simulink subsystem "Control_sub"  (R2023b)
settings: Solver=VariableStepAuto  StartTime=0.0  StopTime=10.0  RelTol=1e-3
libraries: Autonomous_lib x1, Disabled_lib x1, Swerve_Drive_lib x1, Teleop_lib x1, Test_lib x1
settings Model: Creator=USER  LastModifiedBy=USER

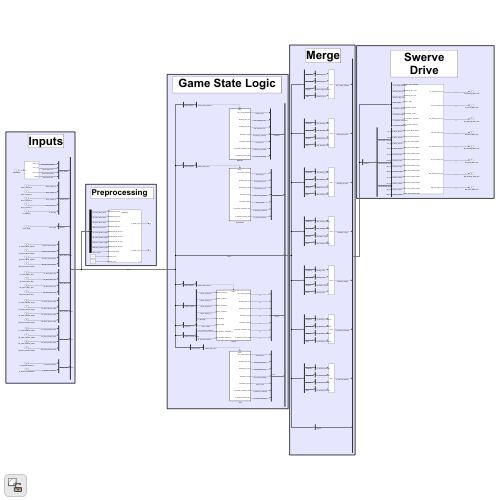
[thumbnail: Simulink's stored preview of the top-level diagram]
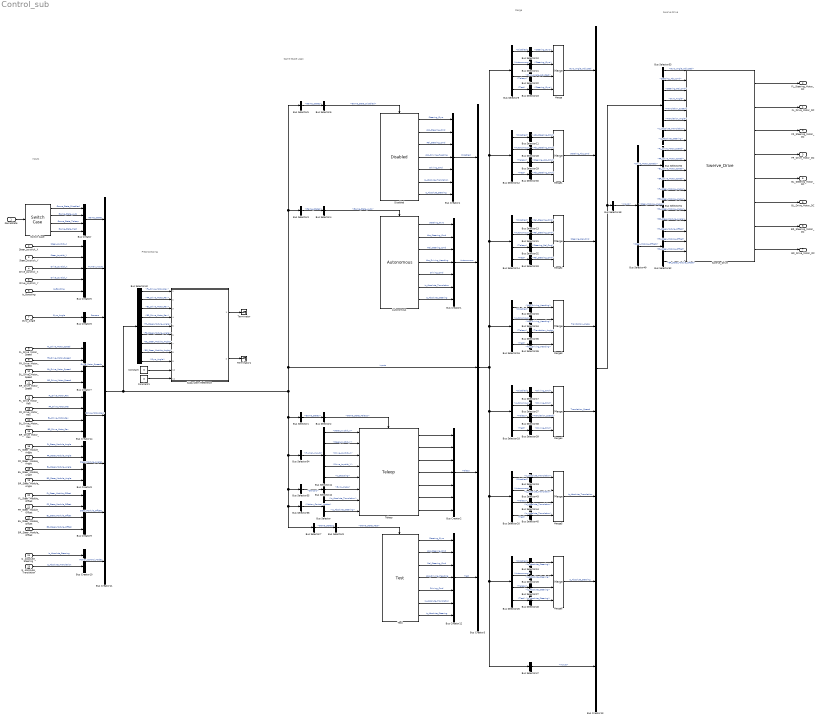
== system Control_sub ==
  note: Game State Logic
  note: Merge
  note: Swerve Drive
  note: Inputs
  note: Preprocessing
  GameState : Inport
  Steer_Joystick_X : Inport  Port=2
  Steer_Joystick_Y : Inport  Port=3
  Drive_Joystick_X : Inport  Port=4
  Drive_Joystick_Y : Inport  Port=5
  Is_Boosting : Inport  Port=6
  Gyro_Angle : Inport  Port=7
  FL_Drive_Motor_Speed : Inport  Port=8
  FR_Drive_Motor_Speed : Inport  Port=9
  BL_Drive_Motor_Speed : Inport  Port=10
  BR_Drive_Motor_Speed : Inport  Port=11
  FL_Drive_Motor_Rev : Inport  Port=12
  FR_Drive_Motor_Rev : Inport  Port=13
  BL_Drive_Motor_Rev : Inport  Port=14
  BR_Drive_Motor_Rev : Inport  Port=15
  FL_Steer_Module_Angle : Inport  Port=16
  FR_Steer_Module_Angle : Inport  Port=17
  BL_Steer_Module_Angle : Inport  Port=18
  BR_Steer_Module_Angle : Inport  Port=19
  FL_Steer_Module_Offset : Inport  Port=20
  FR_Steer_Module_Offset : Inport  Port=21
  BL_Steer_Module_Offset : Inport  Port=22
  BR_Steer_Module_Offset : Inport  Port=23
  Is_Absolute_Steering : Inport  Port=24
  Is_Absolute_Translation : Inport  Port=25
  Autonomous : Autonomous_lib/Autonomous  SystemSampleTime=-1  VariantActivationTime=update diagram  AllowFlexibleInterface=on  Latency=0  AutoFrameSizeCalculation=off
  Bus Creator{,7..9,14} (5 alike) : BusCreator  Inputs=4
  Bus Creator{1..2,4,12} (4 alike) : BusCreator  Inputs=7
  Bus Creator10 : BusCreator  Inputs=2
  Bus Creator11 : BusCreator  Inputs=8
  Bus Creator13 : BusCreator  Inputs=8
  Bus Creator3 : BusCreator  Inputs=5
  Bus Creator5 : BusCreator  Inputs=5
  Bus Creator6 : BusCreator  Inputs=1
  Bus Selector : BusSelector  OutputSignals=Is_Absolute_Translation,Is_Absolute_Steering
  Bus Selector{1,3,5,7} (4 alike) : BusSelector  OutputSignals=Game_States
  Bus Selector10 : BusSelector  OutputSignals=Steering_Gyro
  Bus Selector11 : BusSelector  OutputSignals=Abs_Steering_Cmd
  Bus Selector{9,12,14,16,18,20,25} (7 alike) : BusSelector  OutputSignals=Disabled,Autonomous,Teleop,Test
  Bus Selector13 : BusSelector  OutputSignals=Rel_Steering_Cmd
  Bus Selector15 : BusSelector  OutputSignals=Abs_Driving_Heading
  Bus Selector17 : BusSelector  OutputSignals=Driving_Cmd
  Bus Selector{19,43..45} (4 alike) : BusSelector  OutputSignals=Is_Absolute_Translation
  Bus Selector2 : BusSelector  OutputSignals=Game_State_Teleop
  Bus Selector21 : BusSelector  OutputSignals=Steering_Gyro
  Bus Selector22 : BusSelector  OutputSignals=Gyro_Angle_Adjusted
  Bus Selector23 : BusSelector  OutputSignals=Steering_Gyro
  Bus Selector{24,26..27,46} (4 alike) : BusSelector  OutputSignals=Is_Absolute_Steering
  Bus Selector28 : BusSelector  OutputSignals=Abs_Steering_Cmd
  Bus Selector29 : BusSelector  OutputSignals=Steering_Abs_Cmd
  Bus Selector30 : BusSelector  OutputSignals=Abs_Steering_Cmd
  Bus Selector31 : BusSelector  OutputSignals=Rel_Steering_Cmd
  Bus Selector32 : BusSelector  OutputSignals=Steering_Rel_Cmd
  Bus Selector33 : BusSelector  OutputSignals=Rel_Steering_Cmd
  Bus Selector34 : BusSelector  OutputSignals=Abs_Driving_Heading
  Bus Selector35 : BusSelector  OutputSignals=Translation_Angle
  Bus Selector36 : BusSelector  OutputSignals=Abs_Driving_Heading
  Bus Selector37 : BusSelector  OutputSignals=Driving_Cmd
  Bus Selector38 : BusSelector  OutputSignals=Translation_Speed
  Bus Selector39 : BusSelector  OutputSignals=Driving_Cmd
  Bus Selector4 : BusSelector  OutputSignals=Game_State_Auto
  Bus Selector40 : BusSelector  OutputSignals=Drive_Motor_Revs.FL_Drive_Motor_Rev,Drive_Motor_Revs.FR_Drive_Motor_Rev,Drive_Motor_Revs.BL_Drive_Motor_Rev,Drive_Motor_Revs.BR_Drive_Motor_Rev,Steer_Module_Angles.FL_Steer_Module_Angle,Steer_Module_Angles.FR_Steer_Module_Angle,Steer_Module_Angles.BL_Steer_Module_Angle,Steer_Module_Angles.BR_Steer_Module_Angle,Sensors.Gyro_Angle
  Bus Selector41 : BusSelector  OutputSignals=Steer_Joystick_X,Steer_Joystick_Y,Drive_Joystick_X,Drive_Joystick_Y,Is_Boosting
  Bus Selector42 : BusSelector  OutputSignals=Gyro_Angle
  Bus Selector47 : BusSelector  OutputSignals=Inputs
  Bus Selector48 : BusSelector  OutputSignals=Inputs
  Bus Selector49 : BusSelector  OutputSignals=Drive_Motor_Speeds,Steer_Module_Angles,Steer_Module_Offsets
  Bus Selector50 : BusSelector  OutputSignals=FL_Drive_Motor_Speed,FR_Drive_Motor_Speed,BL_Drive_Motor_Speed,BR_Drive_Motor_Speed
  Bus Selector51 : BusSelector  OutputSignals=FL_Steer_Module_Angle,FR_Steer_Module_Angle,BL_Steer_Module_Angle,BR_Steer_Module_Angle
  Bus Selector52 : BusSelector  OutputSignals=FL_Steer_Module_Offset,FR_Steer_Module_Offset,BL_Steer_Module_Offset,BR_Steer_Module_Offset
  Bus Selector53 : BusSelector  OutputSignals=Gyro_Angle_Adjusted,Steering_Abs_Cmd,Steering_Rel_Cmd,Inputs.Sensors.Gyro_Angle,Translation_Speed,Translation_Angle,Is_Absolute_Translation,Is_Absolute_Steering
  Bus Selector54 : BusSelector  OutputSignals=Human_Inputs
  Bus Selector55 : BusSelector  OutputSignals=Sensors
  Bus Selector56 : BusSelector  OutputSignals=Motion_Control_Modes
  Bus Selector6 : BusSelector  OutputSignals=Game_State_Disabled
  Bus Selector8 : BusSelector  OutputSignals=Game_State_Test
  Constant : Constant  Value=0
  Constant1 : Constant  Value=0
  Disabled : Disabled_lib/Disabled  SystemSampleTime=-1  VariantActivationTime=update diagram  AllowFlexibleInterface=on  Latency=0  AutoFrameSizeCalculation=off
  Merge{,1..6} (7 alike) : Merge  Inputs=4
  Subsystem Reference : Subsystem  ReferencedSubsystem=Odometry
  Swerve_Drive : Swerve_Drive_lib/Swerve_Drive  SystemSampleTime=-1  VariantActivationTime=update diagram  AllowFlexibleInterface=on  Latency=0  AutoFrameSizeCalculation=off
  Switch Case : SwitchCase  CaseConditions={0,1,2}
  Teleop : Teleop_lib/Teleop  SystemSampleTime=-1  VariantActivationTime=update diagram  AllowFlexibleInterface=on  Latency=0  AutoFrameSizeCalculation=off
  Terminator : Terminator
  Terminator1 : Terminator
  Test : Test_lib/Test  SystemSampleTime=-1  VariantActivationTime=update diagram  AllowFlexibleInterface=on  Latency=0  AutoFrameSizeCalculation=off
  FL_Drive_Motor_DC : Outport
  FL_Steering_Motor_DC : Outport  Port=2
  FR_Drive_Motor_DC : Outport  Port=3
  FR_Steering_Motor_DC : Outport  Port=4
  BL_Drive_Motor_DC : Outport  Port=5
  BL_Steering_Motor_DC : Outport  Port=6
  BR_Drive_Motor_DC : Outport  Port=7
  BR_Steering_Motor_DC : Outport  Port=8
  wires:
  Teleop/1 -> Bus Creator2/1
  Teleop/2 -> Bus Creator2/2
  Teleop/3 -> Bus Creator2/3
  Teleop/4 -> Bus Creator2/4
  Teleop/5 -> Bus Creator2/5
  Bus Creator4/1 -> Bus Creator3/1  "Disabled"
  Bus Creator1/1 -> Bus Creator3/2  "Autonomous"
  Bus Creator2/1 -> Bus Creator3/4  "Teleop"
  Switch Case/1 -> Bus Creator/1  "Game_State_Disabled"
  Switch Case/2 -> Bus Creator/2  "Game_State_Auto"
  Switch Case/3 -> Bus Creator/3  "Game_State_Teleop"
  GameState/1 -> Switch Case/1
  Bus Creator12/1 -> Bus Creator3/5  "Test"
  Switch Case/4 -> Bus Creator/4  "Game_State_Test"
  Steer_Joystick_Y/1 -> Bus Creator5/2  "Steer_Joystick_Y"
  Steer_Joystick_X/1 -> Bus Creator5/1  "Steer_Joystick_X"
  Drive_Joystick_X/1 -> Bus Creator5/3  "Drive_Joystick_X"
  Drive_Joystick_Y/1 -> Bus Creator5/4  "Drive_Joystick_Y"
  Gyro_Angle/1 -> Bus Creator6/1  "Gyro_Angle"
  Bus Creator5/1 -> Bus Creator11/2  "Human_Inputs"
  Bus Creator6/1 -> Bus Creator11/3  "Sensors"
  FL_Drive_Motor_Speed/1 -> Bus Creator7/1  "FL_Drive_Motor_Speed"
  FR_Drive_Motor_Speed/1 -> Bus Creator7/2  "FR_Drive_Motor_Speed"
  BL_Drive_Motor_Speed/1 -> Bus Creator7/3  "BL_Drive_Motor_Speed"
  BR_Drive_Motor_Speed/1 -> Bus Creator7/4  "BR_Drive_Motor_Speed"
  FL_Steer_Module_Angle/1 -> Bus Creator8/1  "FL_Steer_Module_Angle"
  BL_Steer_Module_Angle/1 -> Bus Creator8/3  "BL_Steer_Module_Angle"
  BR_Steer_Module_Angle/1 -> Bus Creator8/4  "BR_Steer_Module_Angle"
  FR_Steer_Module_Angle/1 -> Bus Creator8/2  "FR_Steer_Module_Angle"
  Bus Creator7/1 -> Bus Creator11/4  "Drive_Motor_Speeds"
  Bus Creator8/1 -> Bus Creator11/6  "Steer_Module_Angles"
  FL_Steer_Module_Offset/1 -> Bus Creator9/1  "FL_Steer_Module_Offset"
  FR_Steer_Module_Offset/1 -> Bus Creator9/2  "FR_Steer_Module_Offset"
  BL_Steer_Module_Offset/1 -> Bus Creator9/3  "BL_Steer_Module_Offset"
  BR_Steer_Module_Offset/1 -> Bus Creator9/4  "BR_Steer_Module_Offset"
  Bus Creator9/1 -> Bus Creator11/7  "Steer_Module_Offsets"
  Is_Absolute_Steering/1 -> Bus Creator10/1  "Is_Absolute_Steering"
  Is_Absolute_Translation/1 -> Bus Creator10/2  "Is_Absolute_Translation"
  Bus Creator10/1 -> Bus Creator11/8  "Motion_Control_Modes"
  Bus Selector54/1 -> Bus Selector41/1  "<Human_Inputs>"
  Bus Selector41/1 -> Teleop/1  "<Steer_Joystick_X>"
  Bus Selector41/2 -> Teleop/2  "<Steer_Joystick_Y>"
  Bus Selector41/3 -> Teleop/3  "<Drive_Joystick_X>"
  Bus Selector41/4 -> Teleop/4  "<Drive_Joystick_Y>"
  Bus Selector55/1 -> Bus Selector42/1  "<Sensors>"
  Bus Selector42/1 -> Teleop/6  "<Gyro_Angle>"
  Teleop/6 -> Bus Creator2/6
  Teleop/7 -> Bus Creator2/7
  Bus Selector56/1 -> Bus Selector/1  "<Motion_Control_Modes>"
  Bus Selector/2 -> Teleop/8  "<Is_Absolute_Steering>"
  Bus Selector/1 -> Teleop/7  "<Is_Absolute_Translation>"
  Autonomous/2 -> Bus Creator1/2  "Abs_Steering_Cmd"
  Autonomous/4 -> Bus Creator1/4  "Abs_Driving_Heading"
  Autonomous/1 -> Bus Creator1/1  "Steering_Gyro"
  Autonomous/5 -> Bus Creator1/5  "Driving_Cmd"
  Autonomous/7 -> Bus Creator1/7  "Is_Absolute_Steering"
  Autonomous/3 -> Bus Creator1/3  "Rel_Steering_Cmd"
  Autonomous/6 -> Bus Creator1/6  "Is_Absolute_Translation"
  Disabled/2 -> Bus Creator4/2  "Abs_Steering_Cmd"
  Disabled/4 -> Bus Creator4/4  "Abs_Driving_Heading"
  Disabled/1 -> Bus Creator4/1  "Steering_Gyro"
  Disabled/5 -> Bus Creator4/5  "Driving_Cmd"
  Disabled/7 -> Bus Creator4/7  "Is_Absolute_Steering"
  Disabled/3 -> Bus Creator4/3  "Rel_Steering_Cmd"
  Disabled/6 -> Bus Creator4/6  "Is_Absolute_Translation"
  Test/2 -> Bus Creator12/2  "Abs_Steering_Cmd"
  Test/4 -> Bus Creator12/4  "Abs_Driving_Heading"
  Test/1 -> Bus Creator12/1  "Steering_Gyro"
  Test/5 -> Bus Creator12/5  "Driving_Cmd"
  Test/7 -> Bus Creator12/7  "Is_Absolute_Steering"
  Test/3 -> Bus Creator12/3  "Rel_Steering_Cmd"
  Test/6 -> Bus Creator12/6  "Is_Absolute_Translation"
  Bus Creator/1 -> Bus Creator11/1  "Game_States"
  Bus Selector1/1 -> Bus Selector2/1  "<Game_States>"
  Bus Selector2/1 -> Teleop/Action  "<Game_State_Teleop>"
  Bus Selector3/1 -> Bus Selector4/1  "<Game_States>"
  Bus Selector4/1 -> Autonomous/Action  "<Game_State_Auto>"
  Bus Selector5/1 -> Bus Selector6/1  "<Game_States>"
  Bus Selector6/1 -> Disabled/Action  "<Game_State_Disabled>"
  Bus Selector7/1 -> Bus Selector8/1  "<Game_States>"
  Bus Selector8/1 -> Test/Action  "<Game_State_Test>"
  Bus Creator11/1 -> Bus Selector1/1, Bus Selector54/1, Bus Selector55/1, Bus Selector56/1, Bus Selector7/1, Bus Selector3/1, Bus Selector5/1, Bus Creator3/3, Bus Selector40/1  "Inputs"
  Bus Selector9/1 -> Bus Selector10/1  "<Disabled>"
  Bus Selector10/1 -> Merge/1  "<Steering_Gyro>"
  Bus Selector11/1 -> Merge1/1  "<Abs_Steering_Cmd>"
  Bus Selector12/1 -> Bus Selector11/1  "<Disabled>"
  Bus Selector13/1 -> Merge2/1  "<Rel_Steering_Cmd>"
  Bus Selector14/1 -> Bus Selector13/1  "<Disabled>"
  Bus Selector15/1 -> Merge3/1  "<Abs_Driving_Heading>"
  Bus Selector16/1 -> Bus Selector15/1  "<Disabled>"
  Bus Selector17/1 -> Merge4/1  "<Driving_Cmd>"
  Bus Selector18/1 -> Bus Selector17/1  "<Disabled>"
  Bus Selector19/1 -> Merge5/1  "<Is_Absolute_Translation>"
  Bus Selector20/1 -> Bus Selector19/1  "<Disabled>"
  Bus Selector21/1 -> Merge/2  "<Steering_Gyro>"
  Bus Selector9/2 -> Bus Selector21/1  "<Autonomous>"
  Bus Selector22/1 -> Merge/3  "<Gyro_Angle_Adjusted>"
  Bus Selector9/3 -> Bus Selector22/1  "<Teleop>"
  Bus Selector23/1 -> Merge/4  "<Steering_Gyro>"
  Bus Selector9/4 -> Bus Selector23/1  "<Test>"
  Bus Selector25/1 -> Bus Selector24/1  "<Disabled>"
  Bus Selector24/1 -> Merge6/1  "<Is_Absolute_Steering>"
  Bus Creator3/1 -> Bus Selector9/1, Bus Selector12/1, Bus Selector14/1, Bus Selector16/1, Bus Selector18/1, Bus Selector20/1, Bus Selector25/1, Bus Selector47/1
  Bus Selector12/2 -> Bus Selector28/1  "<Autonomous>"
  Bus Selector28/1 -> Merge1/2  "<Abs_Steering_Cmd>"
  Bus Selector12/3 -> Bus Selector29/1  "<Teleop>"
  Bus Selector29/1 -> Merge1/3  "<Steering_Abs_Cmd>"
  Bus Selector12/4 -> Bus Selector30/1  "<Test>"
  Bus Selector30/1 -> Merge1/4  "<Abs_Steering_Cmd>"
  Bus Selector31/1 -> Merge2/2  "<Rel_Steering_Cmd>"
  Bus Selector14/2 -> Bus Selector31/1  "<Autonomous>"
  Bus Selector32/1 -> Merge2/3  "<Steering_Rel_Cmd>"
  Bus Selector14/3 -> Bus Selector32/1  "<Teleop>"
  Bus Selector33/1 -> Merge2/4  "<Rel_Steering_Cmd>"
  Bus Selector14/4 -> Bus Selector33/1  "<Test>"
  Bus Selector16/2 -> Bus Selector34/1  "<Autonomous>"
  Bus Selector34/1 -> Merge3/2  "<Abs_Driving_Heading>"
  Bus Selector16/3 -> Bus Selector35/1  "<Teleop>"
  Bus Selector35/1 -> Merge3/3  "<Translation_Angle>"
  Bus Selector16/4 -> Bus Selector36/1  "<Test>"
  Bus Selector36/1 -> Merge3/4  "<Abs_Driving_Heading>"
  Bus Selector18/2 -> Bus Selector37/1  "<Autonomous>"
  Bus Selector37/1 -> Merge4/2  "<Driving_Cmd>"
  Bus Selector18/3 -> Bus Selector38/1  "<Teleop>"
  Bus Selector38/1 -> Merge4/3  "<Translation_Speed>"
  Bus Selector18/4 -> Bus Selector39/1  "<Test>"
  Bus Selector39/1 -> Merge4/4  "<Driving_Cmd>"
  Bus Selector20/2 -> Bus Selector43/1  "<Autonomous>"
  Bus Selector43/1 -> Merge5/2  "<Is_Absolute_Translation>"
  Bus Selector45/1 -> Merge5/4  "<Is_Absolute_Translation>"
  Bus Selector20/4 -> Bus Selector45/1  "<Test>"
  Bus Selector20/3 -> Bus Selector44/1  "<Teleop>"
  Bus Selector44/1 -> Merge5/3  "<Is_Absolute_Translation>"
  Bus Selector25/2 -> Bus Selector26/1  "<Autonomous>"
  Bus Selector26/1 -> Merge6/2  "<Is_Absolute_Steering>"
  Bus Selector25/4 -> Bus Selector46/1  "<Test>"
  Bus Selector25/3 -> Bus Selector27/1  "<Teleop>"
  Bus Selector46/1 -> Merge6/4  "<Is_Absolute_Steering>"
  Bus Selector27/1 -> Merge6/3  "<Is_Absolute_Steering>"
  Merge/1 -> Bus Creator13/1  "Gyro_Angle_Adjusted"
  Merge1/1 -> Bus Creator13/2  "Steering_Abs_Cmd"
  Merge2/1 -> Bus Creator13/3  "Steering_Rel_Cmd"
  Merge3/1 -> Bus Creator13/4  "Translation_Angle"
  Merge4/1 -> Bus Creator13/5  "Translation_Speed"
  Merge5/1 -> Bus Creator13/6  "Is_Absolute_Translation"
  Merge6/1 -> Bus Creator13/7  "Is_Absolute_Steering"
  Bus Selector47/1 -> Bus Creator13/8  "<Inputs>"
  Bus Creator13/1 -> Bus Selector53/1, Bus Selector48/1
  Bus Selector48/1 -> Bus Selector49/1  "<Inputs>"
  Bus Selector49/1 -> Bus Selector50/1  "<Drive_Motor_Speeds>"
  Bus Selector49/2 -> Bus Selector51/1  "<Steer_Module_Angles>"
  Bus Selector49/3 -> Bus Selector52/1  "<Steer_Module_Offsets>"
  Bus Selector53/1 -> Swerve_Drive/1  "<Gyro_Angle_Adjusted>"
  Bus Selector53/2 -> Swerve_Drive/2  "<Steering_Abs_Cmd>"
  Bus Selector53/3 -> Swerve_Drive/3  "<Steering_Rel_Cmd>"
  Bus Selector53/5 -> Swerve_Drive/5  "<Translation_Speed>"
  Bus Selector53/7 -> Swerve_Drive/7  "<Is_Absolute_Translation>"
  Bus Selector53/8 -> Swerve_Drive/8  "<Is_Absolute_Steering>"
  Bus Selector52/4 -> Swerve_Drive/20  "<BR_Steer_Module_Offset>"
  Bus Selector52/3 -> Swerve_Drive/19  "<BL_Steer_Module_Offset>"
  Bus Selector52/2 -> Swerve_Drive/18  "<FR_Steer_Module_Offset>"
  Bus Selector52/1 -> Swerve_Drive/17  "<FL_Steer_Module_Offset>"
  Bus Selector51/4 -> Swerve_Drive/16  "<BR_Steer_Module_Angle>"
  Bus Selector51/3 -> Swerve_Drive/15  "<BL_Steer_Module_Angle>"
  Bus Selector51/2 -> Swerve_Drive/14  "<FR_Steer_Module_Angle>"
  Bus Selector51/1 -> Swerve_Drive/13  "<FL_Steer_Module_Angle>"
  Bus Selector50/4 -> Swerve_Drive/12  "<BR_Drive_Motor_Speed>"
  Bus Selector50/3 -> Swerve_Drive/11  "<BL_Drive_Motor_Speed>"
  Bus Selector50/2 -> Swerve_Drive/10  "<FR_Drive_Motor_Speed>"
  Bus Selector50/1 -> Swerve_Drive/9  "<FL_Drive_Motor_Speed>"
  Bus Selector53/4 -> Swerve_Drive/4  "<Gyro_Angle>"
  Bus Selector53/6 -> Swerve_Drive/6  "<Translation_Angle>"
  Swerve_Drive/1 -> FL_Steering_Motor_DC/1
  Swerve_Drive/2 -> FL_Drive_Motor_DC/1
  Swerve_Drive/3 -> FR_Steering_Motor_DC/1
  Swerve_Drive/4 -> FR_Drive_Motor_DC/1
  Swerve_Drive/5 -> BL_Steering_Motor_DC/1
  Swerve_Drive/6 -> BL_Drive_Motor_DC/1
  Swerve_Drive/7 -> BR_Steering_Motor_DC/1
  Swerve_Drive/8 -> BR_Drive_Motor_DC/1
  Is_Boosting/1 -> Bus Creator5/5  "Is_Boosting"
  Bus Selector41/5 -> Teleop/5  "<Is_Boosting>"
  Bus Creator14/1 -> Bus Creator11/5  "Drive_Motor_Revs"
  FL_Drive_Motor_Rev/1 -> Bus Creator14/1  "FL_Drive_Motor_Rev"
  FR_Drive_Motor_Rev/1 -> Bus Creator14/2  "FR_Drive_Motor_Rev"
  BL_Drive_Motor_Rev/1 -> Bus Creator14/3  "BL_Drive_Motor_Rev"
  BR_Drive_Motor_Rev/1 -> Bus Creator14/4  "BR_Drive_Motor_Rev"
  Bus Selector40/1 -> Subsystem Reference/1  "<FL_Drive_Motor_Rev>"
  Bus Selector40/2 -> Subsystem Reference/2  "<FR_Drive_Motor_Rev>"
  Bus Selector40/3 -> Subsystem Reference/3  "<BL_Drive_Motor_Rev>"
  Bus Selector40/4 -> Subsystem Reference/4  "<BR_Drive_Motor_Rev>"
  Bus Selector40/5 -> Subsystem Reference/5  "<FL_Steer_Module_Angle>"
  Bus Selector40/6 -> Subsystem Reference/6  "<FR_Steer_Module_Angle>"
  Bus Selector40/7 -> Subsystem Reference/7  "<BL_Steer_Module_Angle>"
  Bus Selector40/8 -> Subsystem Reference/8  "<BR_Steer_Module_Angle>"
  Bus Selector40/9 -> Subsystem Reference/9  "<Gyro_Angle>"
  Constant1/1 -> Subsystem Reference/11
  Constant/1 -> Subsystem Reference/10
  Subsystem Reference/1 -> Terminator/1
  Subsystem Reference/2 -> Terminator1/1
